simulink model "Studio3_31"  (R2017b)
settings: Solver=ode45  StartTime=0.  StopTime=16  FixedStep=0.2  MaxStep=0.05  RelTol=1e-8  AbsTol=1e-8  EnableMultiTasking=on
settings Model: ExtModeTrigMode=oneshot  ExtModeArmWhenConnect=off  Creator=LEVIENKL  LastModifiedBy=carlislt
settings DataIOCC: SaveFormat=Array  SignalLoggingSaveFormat=ModelDataLogs  SaveOutput=off  SaveTime=off  SignalLoggingName=sigsOut
settings OptimizationCC: BlockReduction=off  BooleanDataType=off  ExpressionDepthLimit=2147483647  InitFltsAndDblsToZero=on  LifeSpan=inf
settings DebuggingCC: SaveWithParameterizedLinksMsg=none  UnderspecifiedInitializationDetection=Classic  MergeDetectMultiDrivingBlocksExec=none  SignalResolutionControl=TryResolveAllWithWarning  MultiTaskDSMMsg=warning  MultiTaskCondExecSysMsg=none  FcnCallInpInsideContextMsg=warning  AllowSymbolicDim=off  StateNameClashWarn=warning  SFUnexpectedBacktrackingDiag=warning  SFNoUnconditionalDefaultTransitionDiag=warning  SFExecutionAtInitializationDiag=none
settings HardwareCC: ProdBitPerPointer=32  ProdBitPerSizeT=32  ProdBitPerPtrDiffT=32  ProdLargestAtomicFloat=None  ProdIntDivRoundTo=Undefined  ProdEndianess=Unspecified  ProdWordSize=32  ProdHWDeviceType=32-bit Generic  TargetUnknown=on
settings ModelReferenceCC: PropagateSignalLabelsOutOfModel=off
settings CodeAppCC: StateflowObjectComments=on
settings GRTTargetCC: TargetFcnLib=ansi_tfl_tmw.mat  TargetLangStandard=C89/C90 (ANSI)  GeneratePreprocessorConditionals=Disable all  CombineOutputUpdateFcns=off  GRTInterface=on
settings ConfigComp: CovMetricSettings=dw  CovHtmlReporting=on  CovSaveCumulativeToWorkspaceVar=on  CovSaveSingleToWorkspaceVar=on  CovExternalEMLEnable=off  CovSFcnEnable=off

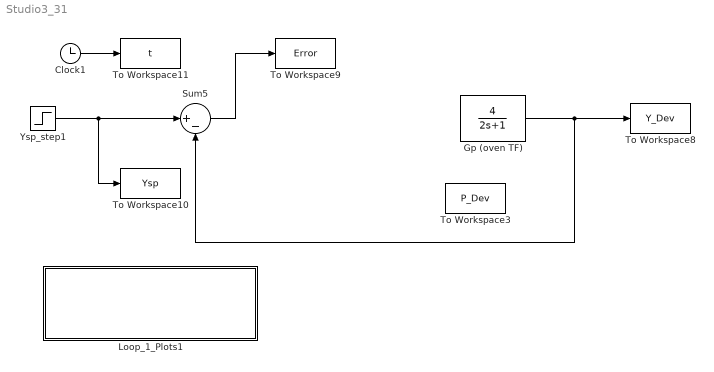
== system Studio3_31 ==
  Clock1 : Clock
  Gp (oven TF) : TransferFcn  Numerator=[4]  Denominator=[2 1]
  Loop_1_Plots1 : Subsystem  mask(Y,U,E Plots - Loop 1){}
      settings: OpenFcn=YPEplots
      mask Help: This block loop #1 Y,U,Error in 3x1 Figure Window.
      mask Display: disp('After Loop 1 Simulation:\n Double Click for Y, P, Error Plots\n (uses YPEplots.p)')
  Sum5 : Sum  Inputs=|+-  SaturateOnIntegerOverflow=on  InputSameDT=on  OutDataTypeStr=Inherit: Same as first input
  To Workspace10 : ToWorkspace  VariableName=Ysp  SampleTime=-1
  To Workspace11 : ToWorkspace  VariableName=t  SampleTime=-1
  To Workspace3 : ToWorkspace  VariableName=P_Dev  SampleTime=-1
  To Workspace8 : ToWorkspace  VariableName=Y_Dev  SampleTime=-1
  To Workspace9 : ToWorkspace  VariableName=Error  SampleTime=-1
  Ysp_step1 : Step  Time=0  After=0  SampleTime=0
      settings: AttributesFormatString=%<Before> to %<After>\nat %<Time>
  wires:
  Clock1/1 -> To Workspace11/1
  Ysp_step1/1 -> To Workspace10/1, Sum5/1
  Sum5/1 -> To Workspace9/1
  Gp (oven TF)/1 -> To Workspace8/1, Sum5/2

== system Studio3_31/Loop_1_Plots1 ==
